simulink model "Arduino_observador"  (R2021a)
settings: Solver=ode4  StartTime=0.0  StopTime=10.0  FixedStep=0.01  RelTol=1e-3  EnableMultiTasking=on
values from neighbouring files (symbols this model uses):
  A = [-Ra/La -Kg/(Kt*La) ... (first row only)    [observador.m]    (also in observador_arduino.m)
  b = [1/La ; 0]    [observador.m]
  c = [0 1]    [observador.m]
  ki_end = valid_ki(end)    [observador.m]
  l = double([sol.l_1;sol.l_2])    [observador.m]
libraries: arduinolib x2
settings Model: SILPILModeSetting=veronly  ExtModeTrigDuration=2  Creator=carol  LastModifiedBy=carol
settings OptimizationCC: EnhancedBackFolding=on  PassReuseOutputArgsAs=Individual arguments  ZeroExternalMemoryAtStartup=off  ZeroInternalMemoryAtStartup=off  MaxStackSize=64  OptimizeBlockOrder=speed  DifferentSizesBufferReuse=on  OptimizationCustomize=off  EfficientTunableParamExpr=on
settings DebuggingCC: ParameterTunabilityLossMsg=error
settings HardwareCC: ProdBitPerPointer=32  ProdBitPerSizeT=32  ProdBitPerPtrDiffT=32  ProdLargestAtomicInteger=Long  ProdLargestAtomicFloat=Double  ProdWordSize=32  ProdHWDeviceType=ARM Compatible->ARM Cortex  UseEmbeddedCoderFeatures=off  UseSimulinkCoderFeatures=off
settings SFSimCC: MATLABDynamicMemAlloc=off
settings RTWCC: SystemTargetFile=ert.tlc  HardwareBoard=Arduino Due  TemplateMakefile=ert_default_tmf  Toolchain=Arduino ARM  BuildConfiguration=Faster Runs
settings CodeAppCC: ForceParamTrailComments=on  IgnoreCustomStorageClasses=off  OperatorAnnotations=on  SimulinkDataObjDesc=on  SFDataObjDesc=on  InsertBlockDesc=on
settings ERTTargetCC: SupportContinuousTime=on  SupportNonInlinedSFcns=on  SupportVariableSizeSignals=on  ExtModeTransport=3  ExtModeStaticAlloc=on  ExtModeStaticAllocSize=24576  ExtModeMexFile=ext_xcp  ExtModeIntrfLevel=Level2 - Open

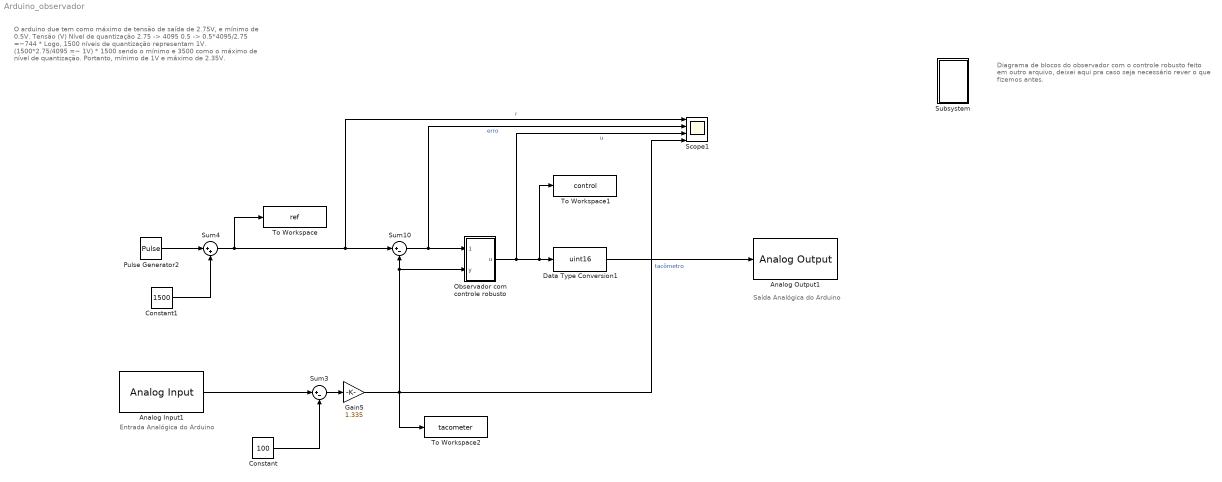
== system Arduino_observador ==
  note: Diagrama de blocos do observador com
      | o controle robusto feito em outro arquivo,
      | deixei aqui pra caso seja necessário rever o
      | que fizemos antes.
  note: Saída Analógica do Arduino
  note: O arduino due tem como máximo de tensão de saída de 2.75V, e mínimo de 0.5V.
      |
      | Tensão (V) Nível de quantização
      | 2.75 -> 4095
      | 0.5 -> 0.5*4095/2.75 =~744
      |
      | * Logo, 1500 níveis de quantização
      | representam 1V.
      | (1500*2.75/4095 =~ 1V)
      |
      | * 1500 sendo o mínimo e 3500 como o máximo de nível de quantização. Portanto,
      | mínimo de 1V e máximo de 2.35V.
  note: Entrada Analógica do Arduino
  Analog Input1 : arduinolib/Analog Input  pinNumber=0  ReadResultsOnly=off  ConversionTriggerSource=Software  ExternalTriggerType=uint32( 0 )  OutputDataType=uint16  EnableConversionCompleteNotify=off  EnableOuputStatus=off  SampleTime=-1  blockPlatform=arduino
  Analog Output1 : arduinolib/Analog Output  DACpin=DAC0  blockPlatform=arduino
      settings: SourceProductBaseCode=ARDUINO
  Constant : Constant  Value=100
  Constant1 : Constant  Value=1500
  Data Type Conversion1 : DataTypeConversion  OutDataTypeStr=uint16
  Gain5 : Gain  Gain=1.335
  Observador com controle robusto : Subsystem
  Pulse Generator2 : DiscretePulseGenerator  PulseType=Time based  Amplitude=2000  Period=3  PulseWidth=50
  Scope1 : Scope  NumInputPorts=4
  Subsystem : Subsystem
  Sum10 : Sum  Inputs=|+-
  Sum3 : Sum  Inputs=|+-
  Sum4 : Sum  Inputs=|++
  To Workspace : ToWorkspace  VariableName=ref  SaveFormat=Structure With Time  SampleTime=-1
  To Workspace1 : ToWorkspace  VariableName=control  SaveFormat=Structure With Time  SampleTime=-1
  To Workspace2 : ToWorkspace  VariableName=tacometer  SaveFormat=Structure With Time  SampleTime=-1
  wires:
  Sum10/1 -> Observador com controle robusto/1(erro), Scope1/2  "erro"
  Sum3/1 -> Gain5/1
  Gain5/1 -> Observador com controle robusto/2(y), Sum10/2, Scope1/4, To Workspace2/1  "tacômetro"
  Observador com controle robusto/1(u) -> Scope1/3, To Workspace1/1, Data Type Conversion1/1  "u"
  Analog Input1/1 -> Sum3/1
  Pulse Generator2/1 -> Sum4/1
  Constant1/1 -> Sum4/2
  Sum4/1 -> Scope1/1, Sum10/1, To Workspace/1  "r"
  Constant/1 -> Sum3/2
  Data Type Conversion1/1 -> Analog Output1/1

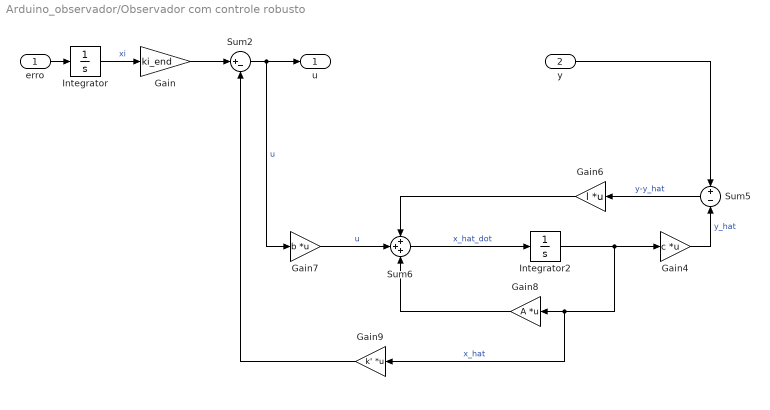
== system Arduino_observador/Observador com controle robusto ==
  erro : Inport
  y : Inport  Port=2
  Gain : Gain  Gain=ki_end
  Gain4 : Gain  Gain=c  Multiplication=Matrix(K*u)
  Gain6 : Gain  Gain=l  Multiplication=Matrix(K*u)
  Gain7 : Gain  Gain=b  Multiplication=Matrix(K*u)
  Gain8 : Gain  Gain=A  Multiplication=Matrix(K*u)
  Gain9 : Gain  Gain=k'  Multiplication=Matrix(K*u)
  Integrator : Integrator
  Integrator2 : Integrator  InitialCondition=6
  Sum2 : Sum  Inputs=|+-
  Sum5 : Sum  Inputs=+|-
  Sum6 : Sum  Inputs=+++
  u : Outport
  wires:
  y/1 -> Sum5/1
  Integrator2/1 -> Gain9/1, Gain8/1, Gain4/1  "x_hat"
  Integrator/1 -> Gain/1  "xi"
  Gain4/1 -> Sum5/2  "y_hat"
  Gain/1 -> Sum2/1
  Sum5/1 -> Gain6/1  "y-y_hat"
  Gain6/1 -> Sum6/1
  Gain9/1 -> Sum2/2
  Gain7/1 -> Sum6/2  "u"
  Gain8/1 -> Sum6/3
  Sum6/1 -> Integrator2/1  "x_hat_dot"
  Sum2/1 -> u/1, Gain7/1  "u"
  erro/1 -> Integrator/1

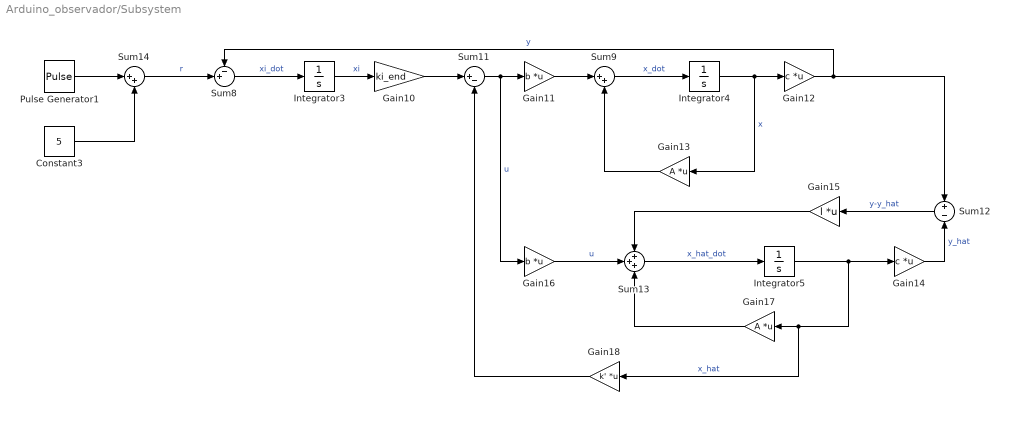
== system Arduino_observador/Subsystem ==
  Constant3 : Constant  Value=5
  Gain10 : Gain  Gain=ki_end
  Gain11 : Gain  Gain=b  Multiplication=Matrix(K*u)
  Gain12 : Gain  Gain=c  Multiplication=Matrix(K*u)
  Gain13 : Gain  Gain=A  Multiplication=Matrix(K*u)
  Gain14 : Gain  Gain=c  Multiplication=Matrix(K*u)
  Gain15 : Gain  Gain=l  Multiplication=Matrix(K*u)
  Gain16 : Gain  Gain=b  Multiplication=Matrix(K*u)
  Gain17 : Gain  Gain=A  Multiplication=Matrix(K*u)
  Gain18 : Gain  Gain=k'  Multiplication=Matrix(K*u)
  Integrator3 : Integrator
  Integrator4 : Integrator  InitialCondition=5
  Integrator5 : Integrator  InitialCondition=6
  Pulse Generator1 : DiscretePulseGenerator  PulseType=Time based  Amplitude=7  PulseWidth=50
  Sum11 : Sum  Inputs=|+-
  Sum12 : Sum  Inputs=+|-
  Sum13 : Sum  Inputs=+++
  Sum14 : Sum  Inputs=|++
  Sum8 : Sum  Inputs=-+|
  Sum9 : Sum  Inputs=|++
  wires:
  Gain18/1 -> Sum11/2
  Gain11/1 -> Sum9/1
  Integrator4/1 -> Gain13/1, Gain12/1  "x"
  Gain14/1 -> Sum12/2  "y_hat"
  Sum8/1 -> Integrator3/1  "xi_dot"
  Gain13/1 -> Sum9/2
  Pulse Generator1/1 -> Sum14/1
  Sum11/1 -> Gain16/1, Gain11/1  "u"
  Gain17/1 -> Sum13/3
  Sum9/1 -> Integrator4/1  "x_dot"
  Gain12/1 -> Sum8/1, Sum12/1  "y"
  Integrator3/1 -> Gain10/1  "xi"
  Sum14/1 -> Sum8/2  "r"
  Constant3/1 -> Sum14/2
  Integrator5/1 -> Gain18/1, Gain17/1, Gain14/1  "x_hat"
  Sum13/1 -> Integrator5/1  "x_hat_dot"
  Gain15/1 -> Sum13/1
  Sum12/1 -> Gain15/1  "y-y_hat"
  Gain16/1 -> Sum13/2  "u"
  Gain10/1 -> Sum11/1
